simulink model "superposition"  (R2022b)
settings: Solver=VariableStepAuto  StartTime=0.0  StopTime=10.0  RelTol=1e-3
libraries: fl_lib x25, nesl_utility x12
settings Model: Creator=saras  LastModifiedBy=saras

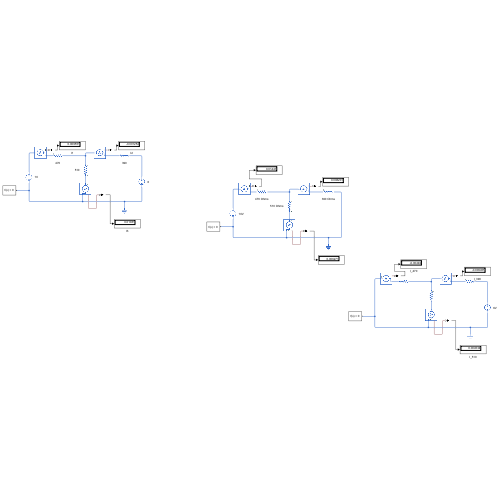
[thumbnail: Simulink's stored preview of the top-level diagram]
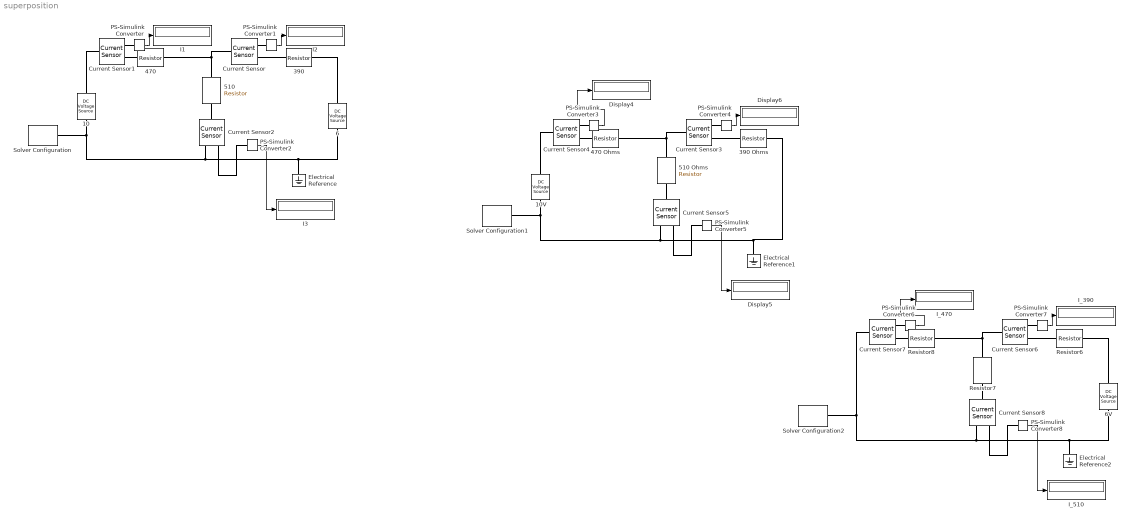
== system superposition ==
  10 : fl_lib/Electrical/Electrical Sources/DC Voltage Source  v0=10 V
  10V : fl_lib/Electrical/Electrical Sources/DC Voltage Source  v0=10 V
  390 : fl_lib/Electrical/Electrical Elements/Resistor  R=390 Ohm  i_specify=on  i_priority=None  i=0 A  i_nominal_specify=on  i_nominal_unit=A  i_nominal_value=1  v_specify=on  v_priority=None  v=0 V  v_nominal_specify=on  v_nominal_unit=V  v_nominal_value=1
  390 Ohms : fl_lib/Electrical/Electrical Elements/Resistor  R=390 Ohm  i_specify=on  i_priority=None  i=0 A  i_nominal_specify=on  i_nominal_unit=A  i_nominal_value=1  v_specify=on  v_priority=None  v=0 V  v_nominal_specify=on  v_nominal_unit=V  v_nominal_value=1
  470 : fl_lib/Electrical/Electrical Elements/Resistor  R=470 Ohm  i_specify=on  i_priority=None  i=0 A  i_nominal_specify=on  i_nominal_unit=A  i_nominal_value=1  v_specify=on  v_priority=None  v=0 V  v_nominal_specify=on  v_nominal_unit=V  v_nominal_value=1
  470 Ohms : fl_lib/Electrical/Electrical Elements/Resistor  R=470 Ohm  i_specify=on  i_priority=None  i=0 A  i_nominal_specify=on  i_nominal_unit=A  i_nominal_value=1  v_specify=on  v_priority=None  v=0 V  v_nominal_specify=on  v_nominal_unit=V  v_nominal_value=1
  510 : fl_lib/Electrical/Electrical Elements/Resistor  R=510 Ohm  i_specify=on  i_priority=None  i=0 A  i_nominal_specify=on  i_nominal_unit=A  i_nominal_value=1  v_specify=on  v_priority=None  v=0 V  v_nominal_specify=on  v_nominal_unit=V  v_nominal_value=1
  510 Ohms : fl_lib/Electrical/Electrical Elements/Resistor  R=510 Ohm  i_specify=on  i_priority=None  i=0 A  i_nominal_specify=on  i_nominal_unit=A  i_nominal_value=1  v_specify=on  v_priority=None  v=0 V  v_nominal_specify=on  v_nominal_unit=V  v_nominal_value=1
  6 : fl_lib/Electrical/Electrical Sources/DC Voltage Source  v0=6 V
  6V : fl_lib/Electrical/Electrical Sources/DC Voltage Source  v0=6 V
  Current Sensor{,1..8} (9 alike) : fl_lib/Electrical/Electrical Sensors/Current Sensor
  Display4 : Display
  Display5 : Display
  Display6 : Display
  Electrical Reference : fl_lib/Electrical/Electrical Elements/Electrical Reference
  Electrical Reference1 : fl_lib/Electrical/Electrical Elements/Electrical Reference
  Electrical Reference2 : fl_lib/Electrical/Electrical Elements/Electrical Reference
  I1 : Display
  I2 : Display
  I3 : Display
  I_390 : Display
  I_470 : Display
  I_510 : Display
  PS-Simulink Converter{,1..8} (9 alike) : nesl_utility/PS-Simulink Converter  PhysicalDomain=network_engine_domain  SubClassName=ps_output  LeftPortType=input  RightPortType=output  PseudoPeriodic=off  Frequencies=[]  VectorFormat=inherit  Unit=inherit  AffineConversion=off
  Resistor6 : fl_lib/Electrical/Electrical Elements/Resistor  R=390 Ohm  i_specify=on  i_priority=None  i=0 A  i_nominal_specify=on  i_nominal_unit=A  i_nominal_value=1  v_specify=on  v_priority=None  v=0 V  v_nominal_specify=on  v_nominal_unit=V  v_nominal_value=1
  Resistor7 : fl_lib/Electrical/Electrical Elements/Resistor  R=510 Ohm  i_specify=on  i_priority=None  i=0 A  i_nominal_specify=on  i_nominal_unit=A  i_nominal_value=1  v_specify=on  v_priority=None  v=0 V  v_nominal_specify=on  v_nominal_unit=V  v_nominal_value=1
  Resistor8 : fl_lib/Electrical/Electrical Elements/Resistor  R=470 Ohm  i_specify=on  i_priority=None  i=0 A  i_nominal_specify=on  i_nominal_unit=A  i_nominal_value=1  v_specify=on  v_priority=None  v=0 V  v_nominal_specify=on  v_nominal_unit=V  v_nominal_value=1
  Solver Configuration : nesl_utility/Solver Configuration  PhysicalDomain=network_engine_domain  SubClassName=solver  LeftPortType=input  RightPortType=generic  Tones=[]  Harmonics=[]  SimulateNoise=off  Profile=off  UseLocalSampling=off  EnableSwitchedLinearOptims=on  FrequencyDomain=off  UseCCode=off  RelTol=0.001  AbsTol=0.001  MinStep=1e-09  ToWorkspace=off  RevertToSquareIcSolve=off  NumHomotopyIterations=100  PhasorMode=off  PhasorModeNumHarmonics=1  ConsistencySolver=NEWTON_XTOL_AFTER_FTOL  IndexReductionMethod=DerivativeReplacement  DoDC=off  ResidualTolerance=1e-09  ConsistencyTolSource=GLOBAL  ConsistencyAbsTol=0.001  ConsistencyRelTol=0.001  ConsistencyTolFactor=0.001  UseLocalSolver=off  LocalSolverChoice=NE_BACKWARD_EULER_ADVANCER  ResolveIndetEquations=on  FunctionEvalNumThread=1  LocalSolverSampleTime=0.001  DoFixedCost=off  MaxNonlinIter=3  MaxModeIter=2  ComputeImpulses=off  ImpulseIterations=2  LinearAlgebra=auto  LinearAlgebraNumThread=0  EquationFormulation=NE_TIME_EF  DelaysMemoryBudget=1024  AutomaticFiltering=on  FilteringTimeConstant=0.001  PartitionStorageMethod=AS_NEEDED  PartitionMemoryBudget=1024  PartitionMethod=ROBUST
  Solver Configuration1 : nesl_utility/Solver Configuration  PhysicalDomain=network_engine_domain  SubClassName=solver  LeftPortType=input  RightPortType=generic  Tones=[]  Harmonics=[]  SimulateNoise=off  Profile=off  UseLocalSampling=off  EnableSwitchedLinearOptims=on  FrequencyDomain=off  UseCCode=off  RelTol=0.001  AbsTol=0.001  MinStep=1e-09  ToWorkspace=off  RevertToSquareIcSolve=off  NumHomotopyIterations=100  PhasorMode=off  PhasorModeNumHarmonics=1  ConsistencySolver=NEWTON_XTOL_AFTER_FTOL  IndexReductionMethod=DerivativeReplacement  DoDC=off  ResidualTolerance=1e-09  ConsistencyTolSource=GLOBAL  ConsistencyAbsTol=0.001  ConsistencyRelTol=0.001  ConsistencyTolFactor=0.001  UseLocalSolver=off  LocalSolverChoice=NE_BACKWARD_EULER_ADVANCER  ResolveIndetEquations=on  FunctionEvalNumThread=1  LocalSolverSampleTime=0.001  DoFixedCost=off  MaxNonlinIter=3  MaxModeIter=2  ComputeImpulses=off  ImpulseIterations=2  LinearAlgebra=auto  LinearAlgebraNumThread=0  EquationFormulation=NE_TIME_EF  DelaysMemoryBudget=1024  AutomaticFiltering=on  FilteringTimeConstant=0.001  PartitionStorageMethod=AS_NEEDED  PartitionMemoryBudget=1024  PartitionMethod=ROBUST
  Solver Configuration2 : nesl_utility/Solver Configuration  PhysicalDomain=network_engine_domain  SubClassName=solver  LeftPortType=input  RightPortType=generic  Tones=[]  Harmonics=[]  SimulateNoise=off  Profile=off  UseLocalSampling=off  EnableSwitchedLinearOptims=on  FrequencyDomain=off  UseCCode=off  RelTol=0.001  AbsTol=0.001  MinStep=1e-09  ToWorkspace=off  RevertToSquareIcSolve=off  NumHomotopyIterations=100  PhasorMode=off  PhasorModeNumHarmonics=1  ConsistencySolver=NEWTON_XTOL_AFTER_FTOL  IndexReductionMethod=DerivativeReplacement  DoDC=off  ResidualTolerance=1e-09  ConsistencyTolSource=GLOBAL  ConsistencyAbsTol=0.001  ConsistencyRelTol=0.001  ConsistencyTolFactor=0.001  UseLocalSolver=off  LocalSolverChoice=NE_BACKWARD_EULER_ADVANCER  ResolveIndetEquations=on  FunctionEvalNumThread=1  LocalSolverSampleTime=0.001  DoFixedCost=off  MaxNonlinIter=3  MaxModeIter=2  ComputeImpulses=off  ImpulseIterations=2  LinearAlgebra=auto  LinearAlgebraNumThread=0  EquationFormulation=NE_TIME_EF  DelaysMemoryBudget=1024  AutomaticFiltering=on  FilteringTimeConstant=0.001  PartitionStorageMethod=AS_NEEDED  PartitionMemoryBudget=1024  PartitionMethod=ROBUST
  wires:
  PS-Simulink Converter/1 -> I1/1
  PS-Simulink Converter1/1 -> I2/1
  PS-Simulink Converter2/1 -> I3/1
  PS-Simulink Converter5/1 -> Display5/1
  PS-Simulink Converter4/1 -> Display6/1
  PS-Simulink Converter3/1 -> Display4/1
  PS-Simulink Converter7/1 -> I_390/1
  PS-Simulink Converter6/1 -> I_470/1
  PS-Simulink Converter8/1 -> I_510/1
  connections:
  470/RConn1 -- 510/LConn1 -- Current Sensor/LConn1
  390/RConn1 -- 6/LConn1
  510/RConn1 -- Current Sensor2/LConn1
  10/RConn1 -- Solver Configuration/RConn1 -- Current Sensor2/RConn2 -- Electrical Reference/LConn1 -- 6/RConn1
  Current Sensor1/LConn1 -- 10/LConn1
  Current Sensor1/RConn2 -- 470/LConn1
  Current Sensor/RConn2 -- 390/LConn1
  PS-Simulink Converter/LConn1 -- Current Sensor1/RConn1
  PS-Simulink Converter1/LConn1 -- Current Sensor/RConn1
  Current Sensor2/RConn1 -- PS-Simulink Converter2/LConn1
  Electrical Reference1/LConn1 -- 390 Ohms/RConn1 -- Solver Configuration1/RConn1 -- 10V/RConn1 -- Current Sensor5/RConn2
  470 Ohms/RConn1 -- 510 Ohms/LConn1 -- Current Sensor3/LConn1
  PS-Simulink Converter3/LConn1 -- Current Sensor4/RConn1
  Current Sensor4/RConn2 -- 470 Ohms/LConn1
  PS-Simulink Converter4/LConn1 -- Current Sensor3/RConn1
  Current Sensor3/RConn2 -- 390 Ohms/LConn1
  Current Sensor5/RConn1 -- PS-Simulink Converter5/LConn1
  Current Sensor4/LConn1 -- 10V/LConn1
  510 Ohms/RConn1 -- Current Sensor5/LConn1
  6V/RConn1 -- Electrical Reference2/LConn1 -- Current Sensor8/RConn2 -- Current Sensor7/LConn1 -- Solver Configuration2/RConn1
  Resistor8/RConn1 -- Resistor7/LConn1 -- Current Sensor6/LConn1
  Current Sensor8/RConn1 -- PS-Simulink Converter8/LConn1
  PS-Simulink Converter7/LConn1 -- Current Sensor6/RConn1
  Resistor6/RConn1 -- 6V/LConn1
  Current Sensor6/RConn2 -- Resistor6/LConn1
  Resistor7/RConn1 -- Current Sensor8/LConn1
  Current Sensor7/RConn2 -- Resistor8/LConn1
  PS-Simulink Converter6/LConn1 -- Current Sensor7/RConn1
